simulink model "taxi_quarc"  (R2025b)
settings: Solver=FixedStepDiscrete  StartTime=0.0  StopTime=inf  FixedStep=0.01  RelTol=1e-3  EnableMultiTasking=on
libraries: quarc_library x2
settings Model: ExtModeTrigDuration=10000  Creator=aguil  LastModifiedBy=aguil
settings SolverCC: AlgebraicLoopSolver=TrustRegion  PositivePriorityOrder=on
settings DataIOCC: ReturnWorkspaceOutputs=off
settings OptimizationCC: LifeSpan=inf
settings DebuggingCC: UnconnectedInputMsg=warning  UnconnectedOutputMsg=warning  UnconnectedLineMsg=warning  ArithmeticOperatorsInVariantConditions=warning
settings ModelReferenceCC: EnableRefExpFcnMdlSchedulingChecks=on
settings SFSimCC: SimUseLocalCustomCode=off  CustomCodeUndefinedFunction=UseInterfaceOnly
settings RTWCC: SystemTargetFile=quarc_win64.tlc  TemplateMakefile=quarc_default_tmf  RTWUseLocalCustomCode=off  GPUComputeCapability=3.5  Description=QUARC Win64 Target
settings CodeAppCC: StateflowObjectComments=on
settings STFCustomTargetCC: SystemTargetFile=quarc_win64.tlc  TargetPreCompLibLocation=C:\PROGRA~3\QUARC\lib\2016a\win64\release  TargetLangStandard=C99 (ISO)  StopOnOverrun=off  Debug=off  DownloadToTarget=on
settings GRTTargetCC: ExtMode=on  ExtModeMexFile=quarc_comm  TargetPreCompLibLocation=C:\PROGRA~3\QUARC\lib\2016a\win64\release  ParMdlRefBuildCompliant=off  CompOptLevelCompliant=off  CombineOutputUpdateFcns=off  MatFileLogging=off  CPPClassGenCompliant=off  GRTInterface=on  UseToolchainInfoCompliant=off
settings ConfigComp: CovMetricSettings=dswe

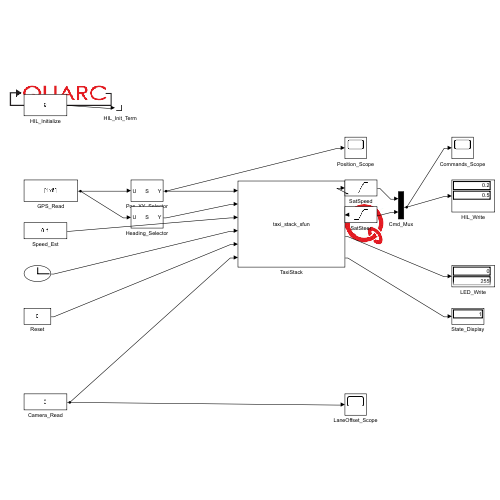
[thumbnail: Simulink's stored preview of the top-level diagram]
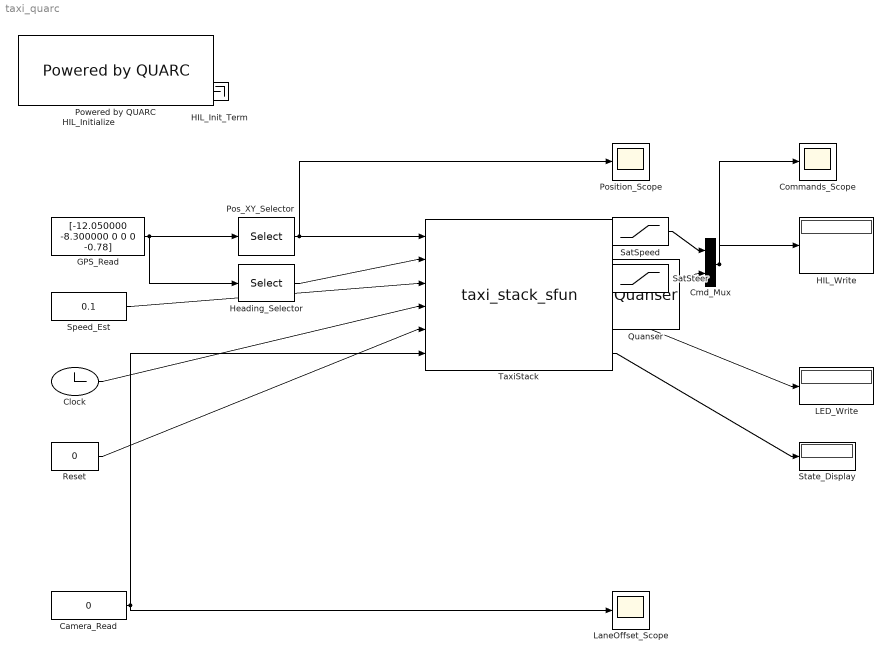
== system taxi_quarc ==
  Camera_Read : Constant  Value=0  OutDataTypeStr=double
  Clock : Clock
  Cmd_Mux : Mux  Inputs=2
  Commands_Scope : Scope
  GPS_Read : Constant  Value=[-12.050000 -8.300000 0 0 0 -0.78]  OutDataTypeStr=double  SampleTime=0.01
  HIL_Init_Term : Terminator
  HIL_Initialize : Constant  Value=0
  HIL_Write : Display
  Heading_Selector : Selector  InputPortWidth=6  IndexOptions=Index vector (dialog)  Indices=6  OutputSizes=1
  LED_Write : Display
  LaneOffset_Scope : Scope
  Pos_XY_Selector : Selector  InputPortWidth=6  IndexOptions=Index vector (dialog)  Indices=[1 2]  OutputSizes=2
  Position_Scope : Scope
  Powered by QUARC : quarc_library/Logos/Powered by QUARC
  Quanser : quarc_library/Logos/Quanser
  Reset : Constant  Value=0
  SatSpeed : Saturate  UpperLimit=0.3  LowerLimit=-0.3
  SatSteer : Saturate
  Speed_Est : Constant  Value=0.1
  State_Display : Display
  TaxiStack : M-S-Function  FunctionName=taxi_stack_sfun
  wires:
  HIL_Initialize/1 -> HIL_Init_Term/1
  GPS_Read/1 -> Pos_XY_Selector/1, Heading_Selector/1
  Pos_XY_Selector/1 -> TaxiStack/1, Position_Scope/1
  Heading_Selector/1 -> TaxiStack/2
  Speed_Est/1 -> TaxiStack/3
  Clock/1 -> TaxiStack/4
  Reset/1 -> TaxiStack/5
  Camera_Read/1 -> TaxiStack/6, LaneOffset_Scope/1
  TaxiStack/1 -> SatSpeed/1
  TaxiStack/2 -> SatSteer/1
  SatSpeed/1 -> Cmd_Mux/1
  SatSteer/1 -> Cmd_Mux/2
  Cmd_Mux/1 -> HIL_Write/1, Commands_Scope/1
  TaxiStack/3 -> LED_Write/1
  TaxiStack/4 -> State_Display/1
